simulink library "fc_vt_lib"  (Simulink 4.00)
undefined symbols (not defined in the file or in its folder): amb_tmp, compressor_mass_flow_map, compressor_pressure_map, compressor_temperature_rise_map, fc_air_comp_scale, fc_allowable_temp_rise, fc_cathode_pressure_drop, fc_cell_area, fc_cell_num, fc_comp_adeff_max, fc_comp_elec_eff, fc_comp_max_tmp, fc_comp_slpm_air_max, fc_comp_spd_max, fc_comp_voleff_max, fc_condenser_fan_flowrate, fc_condenser_fan_num, fc_condenser_fan_pwr_map, fc_condenser_frontal_area, fc_condenser_scale, fc_coolant_pump_flow_map, fc_coolant_pump_pwr_map, fc_cp_air, fc_cp_h2o_l, fc_cp_stack, fc_fuel_lhv, fc_k_air, fc_max_cathode_inlet_pressure, fc_min_cathode_inlet_pressure, fc_min_cell_volts, fc_min_sys_pwr_req, fc_min_temp_for_heat_rejection, fc_mw_air, fc_mw_h2, fc_mw_h20, fc_o2_percent, fc_p_amb, fc_polar_param_concentration, fc_polar_param_ohmic, fc_polar_param_ohmic_temp, fc_polar_param_ref_temp, fc_polar_param_tafel, fc_polar_param_temperature, fc_polar_param_voc, fc_radiator_bypass_delta_t, fc_radiator_fan_flowrate, fc_radiator_fan_num, fc_radiator_fan_pwr_map, fc_radiator_frontal_area, fc_radiator_no_fan_flowrate, fc_radiator_scale, fc_radiator_spd_ratio_fan_off, fc_radiator_spd_ratio_fan_on, fc_radiator_veh_spd_map, fc_reference_temperature, fc_rh_amb, fc_stack_i_map, fc_stack_pres_cor_map, fc_stack_pres_map, fc_stack_stoich_air_map ... (+10)
libraries: fc_vt_lib x54, simulink3 x9
(part 2 of 3)

== system fc_vt_lib/VT_FUELCELL_MODEL ==
  net Power Request : Inport  Port=1  LatchInput=off
  Constant2 : Constant  Value=fc_min_sys_pwr_req
  Demux : Demux  Outputs=6  BusSelectionMode=off
  If : If  NumInputs=2  IfExpression=u1<u2  ShowElse=on
  Mux2 : Mux  Orientation=left  Inputs=4
  Subsystem : Subsystem
      settings: RTWFcnNameOpts=Auto  RTWFileNameOpts=Auto
  Switch : Switch  Threshold=1
  Terminator : Terminator
  Water : Memory  Orientation=left  X0=0  InheritSampleTime=off
      settings: RTWStateStorageClass=Auto
  min_cell_voltage & net power gen : Subsystem  TreatAsAtomicUnit=on
      settings: RTWFcnNameOpts=Auto  RTWFileNameOpts=Auto
  min_system_power : Subsystem  TreatAsAtomicUnit=on
      settings: RTWFcnNameOpts=Auto  RTWFileNameOpts=Auto
  stack_temperature : Memory  Orientation=left  X0=fc_system_init_temp  InheritSampleTime=off
      settings: RTWStateStorageClass=Auto
  t_stack_coolant_in : Memory  Orientation=left  X0=fc_system_init_temp  InheritSampleTime=off
      settings: RTWStateStorageClass=Auto
  Net Power Gen : Outport  Port=1
  system_characteristics : Outport  Port=2
  wires:
  Demux/1 -> Net Power Gen/1
  Demux/2 -> stack_temperature/1
  Demux/4 -> t_stack_coolant_in/1
  Demux/5 -> Water/1
  t_stack_coolant_in/1 -> Mux2/2
  stack_temperature/1 -> Mux2/3
  Water/1 -> Mux2/4
  Subsystem/1(system_characteristics) -> system_characteristics/1
  Demux/6 -> Subsystem/1(In1)
  [net_power_request] -> If/1
  Constant2/1 -> If/2
  [net_power_request] -> Mux2/1
  Mux2/1 -> [system_input]
  [system_input] -> min_system_power/1(In1)
  If/2 -> min_cell_voltage & net power gen/Action
  [system_input] -> min_cell_voltage & net power gen/1(In1)
  If/1 -> min_system_power/Action
  min_system_power/1(system_characteristics) -> Switch/1
  min_system_power/2(enabled?) -> Switch/2
  min_cell_voltage & net power gen/1(Out1) -> Switch/3
  Switch/1 -> Demux/1
  net Power Request/1 -> [net_power_request]
  Demux/3 -> Terminator/1

== system fc_vt_lib/air_power ==
  note: [K]
  m_dot_air : Inport  Port=1  LatchInput=off
  eff_overall : Inport  Port=2  LatchInput=off
  pressure : Inport  Port=3  LatchInput=off
  Constant : Constant  Value=amb_tmp
  Constant1 : Constant  Value=fc_k_air
  Constant2 : Constant  Value=fc_k_air
  Constant3 : Constant  Value=1
  Constant5 : Constant  Value=1
  Constant6 : Constant  Value=fc_comp_elec_eff
  Cp Air : fc_vt_lib/Cp Water_Vapor
      settings: RTWFcnNameOpts=Auto  RTWFileNameOpts=Auto
  Math Function : Math  Operator=pow  OutputSignalType=auto
  Product : Product  Inputs=4  Multiplication=Element-wise(.*)  SaturateOnIntegerOverflow=on
  Product1 : Product  Inputs=*/  Multiplication=Element-wise(.*)  SaturateOnIntegerOverflow=on
  Product2 : Product  Inputs=*//  Multiplication=Element-wise(.*)  SaturateOnIntegerOverflow=on
  Sum : Sum  Inputs=|+-  SaturateOnIntegerOverflow=on
  Sum1 : Sum  Inputs=|+-  SaturateOnIntegerOverflow=on
  Sum2 : Sum  Inputs=|++  SaturateOnIntegerOverflow=on
  const : Constant  Value=273.15
  Out1 : Outport  Port=1
  wires:
  Cp Air/1 -> Product/2
  Product2/1 -> Out1/1
  eff_overall/1 -> Product2/3
  Constant6/1 -> Product2/2
  Product/1 -> Product2/1
  Sum1/1 -> Product/4
  Math Function/1 -> Sum1/1
  Constant5/1 -> Sum1/2
  Product1/1 -> Math Function/2
  pressure/1 -> Math Function/1
  Constant2/1 -> Product1/2
  Sum/1 -> Product1/1
  Constant3/1 -> Sum/2
  Constant1/1 -> Sum/1
  m_dot_air/1 -> Product/1
  Sum2/1 -> Cp Air/1, Product/3
  Constant/1 -> Sum2/2
  const/1 -> Sum2/1

== system fc_vt_lib/h2W ==
  temp : Inport  Port=1  LatchInput=off
  pressure (atm) : Inport  Port=2  LatchInput=off
  rh : Inport  Port=3  LatchInput=off
  1=air;  2=h2 : Inport  Port=4  LatchInput=off
  Constant : Constant  Value=fc_mw_h20
  Constant1 : Constant  Value=fc_mw_air
  Constant2 : Constant  Value=fc_mw_h2
  Product : Product  Inputs=*/*/  Multiplication=Element-wise(.*)  SaturateOnIntegerOverflow=on
  Product1 : Product  Inputs=2  Multiplication=Element-wise(.*)  SaturateOnIntegerOverflow=on
  Psat : fc_vt_lib/Psat
      settings: RTWFcnNameOpts=Auto  RTWFileNameOpts=Auto
  Sum : Sum  Inputs=-+  SaturateOnIntegerOverflow=on
  Switch : Switch  Threshold=2
  atm --> kPa : Gain  Gain=101.325  Multiplication=Element-wise(K.*u)  SaturateOnIntegerOverflow=on
  w : Outport  Port=1
  wires:
  Constant/1 -> Product/1
  temp/1 -> Psat/1
  Psat/1 -> Product1/1
  pressure (atm)/1 -> atm --> kPa/1
  rh/1 -> Product1/2
  Product1/1 -> Sum/1, Product/3
  Sum/1 -> Product/4
  Constant2/1 -> Switch/1
  1=air;  2=h2/1 -> Switch/2
  Constant1/1 -> Switch/3
  Switch/1 -> Product/2
  Product/1 -> w/1
  atm --> kPa/1 -> Sum/2

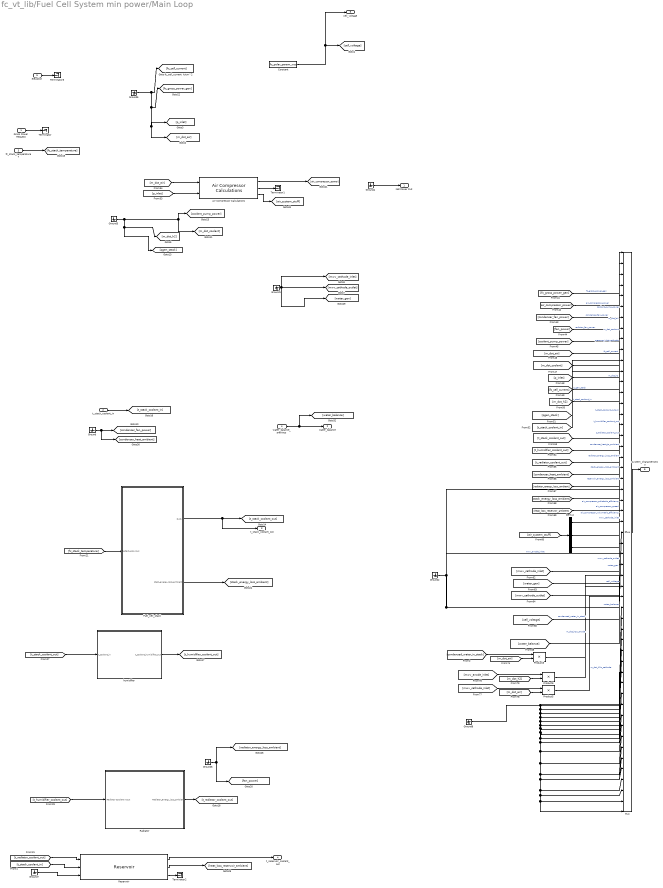
== system fc_vt_lib/Fuel Cell System min power/Main Loop ==
  Gross Power Request : Inport  Port=1  LatchInput=off
  t_stack_coolant_in : Inport  Port=2  LatchInput=off
  fc_stack_temperature7 : Inport  Port=3  LatchInput=off
  water_balance_previous : Inport  Port=4  LatchInput=off
  elevation : Inport  Port=5  LatchInput=off
  Air Compressor Calculations : fc_vt_lib/Main Loop/Air Compressor Calculations
      settings: RTWFcnNameOpts=Auto  RTWFileNameOpts=Auto
  Constant : Constant  Value=fc_polar_param_voc
  Demux : Demux  Outputs=3  BusSelectionMode=off
  Fuel_cell_stack : Subsystem  AncestorBlock=fc_vt_lib/Fuel Cell System min power/Main Loop/Fuel_cell_stack
      settings: RTWFcnNameOpts=Auto  RTWFileNameOpts=Auto
  Ground{,1..8} (9 alike) : Ground
  Mux : Mux  Inputs=53
  Product3 : Product  Inputs=2  Multiplication=Element-wise(.*)  SaturateOnIntegerOverflow=on
  Product5 : Product  Inputs=2  Multiplication=Element-wise(.*)  SaturateOnIntegerOverflow=on
  Product6 : Product  Inputs=2  Multiplication=Element-wise(.*)  SaturateOnIntegerOverflow=on
  Radiator : Subsystem  AncestorBlock=fc_vt_lib/Fuel Cell System min power/Main Loop/Radiator
      settings: RTWFcnNameOpts=Auto  RTWFileNameOpts=Auto
  Reservoir : fc_vt_lib/Main Loop/Reservoir
      settings: RTWFcnNameOpts=Auto  RTWFileNameOpts=Auto
  Terminator{,1..3} (4 alike) : Terminator
  humidifier : Subsystem  AncestorBlock=fc_vt_lib/Fuel Cell System min power/Main Loop/humidifier
      settings: RTWFcnNameOpts=Auto  RTWFileNameOpts=Auto
  Net Power Out : Outport  Port=1
  water_balance : Outport  Port=2
  t_stack_coolant_out : Outport  Port=3
  t_reservoir_coolant_out : Outport  Port=4
  cell_voltage : Outport  Port=5
  system_characteristics : Outport  Port=6
  wires:
  Air Compressor Calculations/2 -> Terminator1/1
  Ground3/1 -> [m_dot_coolant], [coolant_pump_power], [m_dot_h2], [qgen_stack]
  Ground4/1 -> Net Power Out/1
  [water_balance] -> Mux/30  "water_balance"
  [cell_voltage] -> Mux/28  "cell_voltage"
  Ground2/1 -> Mux/23, Mux/27, Mux/29  "mwv_anode_inlet"
  [mwv_cathode_inlet] -> Mux/24  "mwv_cathode_inlet"
  [water_gen] -> Mux/25  "water_gen"
  [mwv_cathode_outlet] -> Mux/26  "mwv_cathode_outlet"
  t_stack_coolant_in/1 -> [t_stack_coolant_in]
  fc_stack_temperature7/1 -> [fc_stack_temperature]
  [t_humidifier_coolant_out] -> Radiator/1(Radiator Coolant Input)
  Constant/1 -> [cell_voltage], cell_voltage/1
  Ground1/1 -> [mwv_cathode_inlet], [mwv_cathode_outlet], [water_gen]
  [t_radiator_coolant_out] -> Reservoir/1
  Reservoir/1 -> t_reservoir_coolant_out/1
  [t_stack_coolant_out] -> humidifier/1(t_coolant_in)
  humidifier/1(t_coolant_humidifier_out) -> [t_humidifier_coolant_out]
  [fc_stack_temperature] -> Fuel_cell_stack/1(t_stack_previous)
  Fuel_cell_stack/1(Out1) -> t_stack_coolant_out/1, [t_stack_coolant_out]
  Fuel_cell_stack/2(stack_energy_loss_ambient) -> [stack_energy_loss_ambient]
  Reservoir/2 -> [heat_loss_reservoir_ambient]
  Demux/3 -> Mux/22  "air_compressor_volumetric_efficiency"
  Demux/2 -> Mux/21  "air_compressor_adiabatic_efficiency"
  Demux/1 -> Mux/20  "air_compressor_speed"
  [heat_loss_reservoir_ambient] -> Mux/19  "reservoir_energy_loss_ambient"
  [stack_energy_loss_ambient] -> Mux/18  "stack_energy_loss_ambient"
  [radiator_energy_loss_ambient] -> Mux/17  "radiator_energy_loss_ambient"
  [condenser_heat_ambient] -> Mux/16  "condenser_heat_to_ambient"
  [t_radiator_coolant_out] -> Mux/15  "t_radiator_coolant_out"
  [t_humidifier_coolant_out] -> Mux/14  "t_humidifier_coolant_out"
  [t_stack_coolant_out] -> Mux/13  "t_stack_coolant_output"
  [t_stack_coolant_in] -> Mux/12  "t_stack_coolant_in"
  [qgen_stack] -> Mux/11  "q_gen_stack"
  [m_dot_h2] -> Mux/10  "m_dot_h2"
  [fc_cell_current] -> Mux/9  "fc_cell_current"
  [p_inlet] -> Mux/8  "pressure_inlet_cathode"
  [m_dot_coolant] -> Mux/7  "m_dot_coolant"
  [m_dot_air] -> Mux/6  "m_dot_air"
  [coolant_pump_power] -> Mux/5  "coolant_pump_power"
  [fan_power] -> Mux/4  "radiator_fan_power"
  [condenser_fan_power] -> Mux/3  "condenser_fan_power"
  [air_compressor_power] -> Mux/2  "air_compressor_power"
  [fc_gross_power_gen] -> Mux/1  "fc_gross_power_gen"
  [air_system_stuff] -> Demux/1
  Mux/1 -> system_characteristics/1
  Ground/1 -> [condenser_fan_power], [condenser_heat_ambient]
  [p_inlet] -> Air Compressor Calculations/2
  [m_dot_air] -> Air Compressor Calculations/1
  Air Compressor Calculations/1 -> [air_compressor_power]
  Air Compressor Calculations/3 -> [air_system_stuff]
  Ground5/1 -> [fc_cell_current], [fc_gross_power_gen], [p_inlet], [m_dot_air]
  Gross Power Request/1 -> Terminator/1
  Ground6/1 -> [fan_power], [radiator_energy_loss_ambient]
  Radiator/1(Radiator_energy_loss_ambient) -> [t_radiator_coolant_out]
  Ground7/1 -> Reservoir/3
  [t_stack_coolant_in] -> Reservoir/2
  Reservoir/3 -> Terminator2/1
  water_balance_previous/1 -> water_balance/1, [water_balance]
  Product3/1 -> Mux/31  "condensed_water_in_stack"
  [mwv_cathode_inlet] -> Product5/1
  [m_dot_air] -> Product5/2
  [mwv_anode_inlet] -> Product6/1
  [m_dot_h2] -> Product6/2
  Product6/1 -> Mux/32  "m_dot_h2o_anode"
  Product5/1 -> Mux/33  "m_dot_h2o_cathode"
  [condensed_water_in_stack] -> Product3/1
  [m_dot_air] -> Product3/2
  Ground8/1 -> Mux/41, Mux/42, Mux/43, Mux/44, Mux/45, Mux/46, Mux/47, Mux/48, Mux/49, Mux/50, Mux/51, Mux/52, Mux/53, Mux/40, Mux/39, Mux/38, Mux/37, Mux/36, Mux/35, Mux/34
  elevation/1 -> Terminator3/1

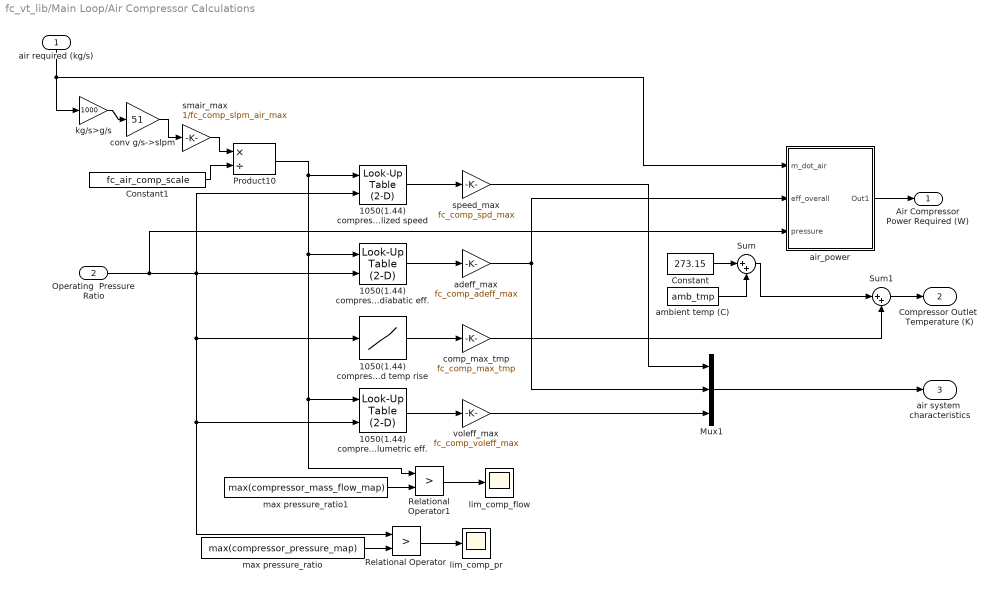
== system fc_vt_lib/Main Loop/Air Compressor Calculations ==
  " air required (kg/s)" : Inport  Orientation=down  Port=1  LatchInput=off
  Operating  Pressure Ratio : Inport  Port=2  LatchInput=off
  1050(1.44) compressor normalized adiabatic eff. : simulink3/Functions & Tables/Look-Up Table (2-D)  x=compressor_mass_flow_map  y=compressor_pressure_map  t=CC
  1050(1.44) compressor normalized speed : simulink3/Functions & Tables/Look-Up Table (2-D)  x=compressor_mass_flow_map  y=compressor_pressure_map  t=BB
  1050(1.44) compressor normalized temp rise : Lookup  InputValues=compressor_pressure_map  OutputValues=compressor_temperature_rise_map
  1050(1.44) compressor normalized volumetric eff. : simulink3/Functions & Tables/Look-Up Table (2-D)  x=compressor_mass_flow_map  y=compressor_pressure_map  t=DD
  Constant : Constant  Value=273.15
  Constant1 : Constant  Value=fc_air_comp_scale
  Mux1 : Mux  Inputs=3
  Product10 : Product  Inputs=*/  Multiplication=Element-wise(.*)  SaturateOnIntegerOverflow=on
  Relational Operator : RelationalOperator  Operator=>
  Relational Operator1 : RelationalOperator  Operator=>
  Sum : Sum  Inputs=|++  SaturateOnIntegerOverflow=on
  Sum1 : Sum  Inputs=|++  SaturateOnIntegerOverflow=on
  adeff_max : Gain  Gain=fc_comp_adeff_max  Multiplication=Element-wise(K.*u)  SaturateOnIntegerOverflow=on
  air_power : Subsystem  AncestorBlock=fc_vt_lib/air_power
      settings: RTWFcnNameOpts=Auto  RTWFileNameOpts=Auto
  ambient temp (C) : Constant  Value=amb_tmp
  comp_max_tmp : Gain  Gain=fc_comp_max_tmp  Multiplication=Element-wise(K.*u)  SaturateOnIntegerOverflow=on
  conv g/s->slpm : Gain  Gain=51  Multiplication=Element-wise(K.*u)  SaturateOnIntegerOverflow=on
  kg/s>g/s : Gain  Gain=1000  Multiplication=Element-wise(K.*u)  SaturateOnIntegerOverflow=on
  lim_comp_flow : Scope
      settings: TimeRange=auto  YMin=-5  YMax=5  SaveToWorkspace=off  LimitDataPoints=on  MaxDataPoints=5000
  lim_comp_pr : Scope
      settings: TimeRange=auto  YMin=-5  YMax=5  SaveToWorkspace=off  SaveName=ScopeData  LimitDataPoints=on  MaxDataPoints=5000
  max pressure_ratio : Constant  Value=max(compressor_pressure_map)
  max pressure_ratio1 : Constant  Value=max(compressor_mass_flow_map)
  smair_max : Gain  Gain=1/fc_comp_slpm_air_max  Multiplication=Element-wise(K.*u)  SaturateOnIntegerOverflow=on
  speed_max : Gain  Gain=fc_comp_spd_max  Multiplication=Element-wise(K.*u)  SaturateOnIntegerOverflow=on
  voleff_max : Gain  Gain=fc_comp_voleff_max  Multiplication=Element-wise(K.*u)  SaturateOnIntegerOverflow=on
  Air Compressor Power Required (W) : Outport  Port=1
  Compressor Outlet  Temperature (K) : Outport  Port=2
  air system  characteristics : Outport  Port=3
  wires:
  1050(1.44) compressor normalized volumetric eff./1 -> voleff_max/1
  comp_max_tmp/1 -> Sum1/2
  1050(1.44) compressor normalized temp rise/1 -> comp_max_tmp/1
  1050(1.44) compressor normalized adiabatic eff./1 -> adeff_max/1
  1050(1.44) compressor normalized speed/1 -> speed_max/1
  conv g/s->slpm/1 -> smair_max/1
  adeff_max/1 -> Mux1/2, air_power/2(eff_overall)
  " air required (kg/s)"/1 -> air_power/1(m_dot_air), kg/s>g/s/1
  Operating  Pressure Ratio/1 -> air_power/3(pressure), 1050(1.44) compressor normalized temp rise/1, 1050(1.44) compressor normalized volumetric eff./2, Relational Operator/1, 1050(1.44) compressor normalized speed/2, 1050(1.44) compressor normalized adiabatic eff./2
  Sum1/1 -> Compressor Outlet  Temperature (K)/1
  speed_max/1 -> Mux1/1
  voleff_max/1 -> Mux1/3
  Mux1/1 -> air system  characteristics/1
  air_power/1(Out1) -> Air Compressor Power Required (W)/1
  Constant/1 -> Sum/1
  ambient temp (C)/1 -> Sum/2
  Sum/1 -> Sum1/1
  max pressure_ratio/1 -> Relational Operator/2
  Relational Operator/1 -> lim_comp_pr/1
  max pressure_ratio1/1 -> Relational Operator1/2
  Relational Operator1/1 -> lim_comp_flow/1
  smair_max/1 -> Product10/1
  Product10/1 -> 1050(1.44) compressor normalized speed/1, 1050(1.44) compressor normalized adiabatic eff./1, 1050(1.44) compressor normalized volumetric eff./1, Relational Operator1/1
  Constant1/1 -> Product10/2
  kg/s>g/s/1 -> conv g/s->slpm/1

== system fc_vt_lib/Main Loop/Air Requirement Calculation ==
  Cell Voltage (V) : Inport  Port=1  LatchInput=off
  Fuel Cell Gross Power (W) : Inport  Port=2  LatchInput=off
  Stoic Rate Air : Inport  Port=3  LatchInput=off
  %-->fraction : Gain  Gain=1/100  Multiplication=Element-wise(K.*u)  SaturateOnIntegerOverflow=on
  4*F : Constant  Value=4*96485
  Molecular Weight of  Inlet Air (g/mole) : Subsystem
      settings: RTWFcnNameOpts=Auto  RTWFileNameOpts=Auto
  Molecular weight  of N2 (g/mole) : Constant  Value=28
  O2 Molecular Weight  (g/mole) : Constant  Value=32
  Product : Product  Inputs=**//  Multiplication=Element-wise(.*)  SaturateOnIntegerOverflow=on
  Product1 : Product  Inputs=*/*  Multiplication=Element-wise(.*)  SaturateOnIntegerOverflow=on
  g/s-->kg/s : Gain  Gain=1/1000  Multiplication=Element-wise(K.*u)  SaturateOnIntegerOverflow=on
  percent O2 in air : Constant  Value=fc_o2_percent
  m_dot_air kg/s : Outport  Port=1
  wires:
  O2 Molecular Weight  (g/mole)/1 -> Molecular Weight of  Inlet Air (g/mole)/2(In2)
  Stoic Rate Air/1 -> Product/1
  4*F/1 -> Product/4
  percent O2 in air/1 -> %-->fraction/1
  %-->fraction/1 -> Molecular Weight of  Inlet Air (g/mole)/1(In1), Product1/2
  Molecular Weight of  Inlet Air (g/mole)/1(Out1) -> Product1/3
  g/s-->kg/s/1 -> m_dot_air kg/s/1
  Product1/1 -> g/s-->kg/s/1
  Product/1 -> Product1/1
  Fuel Cell Gross Power (W)/1 -> Product/2
  Cell Voltage (V)/1 -> Product/3
  Molecular weight  of N2 (g/mole)/1 -> Molecular Weight of  Inlet Air (g/mole)/3(In3)

== system fc_vt_lib/Main Loop/Calculate the Required Water Flowrate for the Pump ==
  Stack gross Power Gen : Inport  Port=1  LatchInput=off
  Cell Voltage : Inport  Port=2  LatchInput=off
  2*F : Constant  Value=2*96485
  Deg C Rise : Constant  Value=fc_allowable_temp_rise
  J/g-->J/kg : Gain  Gain=1000  Multiplication=Element-wise(K.*u)  SaturateOnIntegerOverflow=on
  Lower Heating Value  Hydrogen (J/g) : Constant  Value=fc_fuel_lhv
  Molecular Weight H2  (kg/mole) : Constant  Value=2.02/1000
  Product : Product  Inputs=2  Multiplication=Element-wise(.*)  SaturateOnIntegerOverflow=on
  Product1 : Product  Inputs=*//  Multiplication=Element-wise(.*)  SaturateOnIntegerOverflow=on
  Specific Heat Water : Constant  Value=fc_cp_h2o_l
  Sum1 : Sum  Inputs=+-  SaturateOnIntegerOverflow=on
  m_dot_h2 : Product  Inputs=**//  Multiplication=Element-wise(.*)  SaturateOnIntegerOverflow=on
  coolant (kg/s) : Outport  Port=1
  m_dot_hydrogen : Outport  Port=2
  q_gen_stack : Outport  Port=3
  wires:
  Stack gross Power Gen/1 -> Sum1/2, m_dot_h2/1
  m_dot_h2/1 -> Product/1, m_dot_hydrogen/1
  Lower Heating Value  Hydrogen (J/g)/1 -> J/g-->J/kg/1
  Product/1 -> Sum1/1
  Sum1/1 -> Product1/1, q_gen_stack/1
  Deg C Rise/1 -> Product1/2
  Specific Heat Water/1 -> Product1/3
  Cell Voltage/1 -> m_dot_h2/3
  Product1/1 -> coolant (kg/s)/1
  Molecular Weight H2  (kg/mole)/1 -> m_dot_h2/2
  J/g-->J/kg/1 -> Product/2
  2*F/1 -> m_dot_h2/4

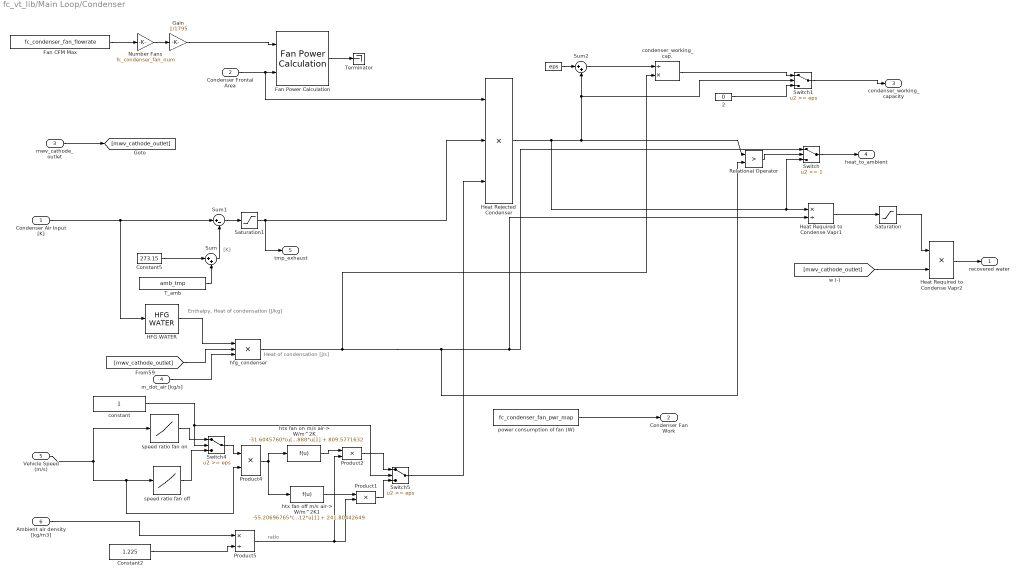
== system fc_vt_lib/Main Loop/Condenser ==
  note: [K]
  note: Enthalpy, Heat of condensation [J/kg]
  note: Heat of condensation [J/s]
  note: ratio
  Condenser Air Input [K] : Inport  Port=1  LatchInput=off
  Condenser Frontal Area : Inport  Port=2  LatchInput=off
  mwv_cathode_outlet : Inport  Port=3  LatchInput=off
  m_dot_air [kg/s] : Inport  Port=4  LatchInput=off
  Vehicle Speed (m/s) : Inport  Port=5  LatchInput=off
  Ambient air density [kg/m3] : Inport  Port=6  LatchInput=off
  " " : Constant  Value=eps
  " 2" : Constant  Value=0
  Constant2 : Constant  Value=1.225
  Constant5 : Constant  Value=273.15
  Fan CFM Max : Constant  Value=fc_condenser_fan_flowrate
  Fan Power Calculation : fc_vt_lib/Fan Power Calculation
      settings: RTWFcnNameOpts=Auto  RTWFileNameOpts=Auto
  Gain : Gain  Gain=1/1795  Multiplication=Element-wise(K.*u)  SaturateOnIntegerOverflow=on
  HFG WATER : fc_vt_lib/HFG WATER
      settings: RTWFcnNameOpts=Auto  RTWFileNameOpts=Auto
  Heat Rejected Condenser : Product  Inputs=***  Multiplication=Element-wise(.*)  SaturateOnIntegerOverflow=on
  Heat Required to Condense Vapr1 : Product  Inputs=*/  Multiplication=Element-wise(.*)  SaturateOnIntegerOverflow=on
  Heat Required to Condense Vapr2 : Product  Inputs=**  Multiplication=Element-wise(.*)  SaturateOnIntegerOverflow=on
  Number Fans : Gain  Gain=fc_condenser_fan_num  Multiplication=Element-wise(K.*u)  SaturateOnIntegerOverflow=on
  Product1 : Product  Inputs=**  Multiplication=Element-wise(.*)  SaturateOnIntegerOverflow=on
  Product2 : Product  Inputs=**  Multiplication=Element-wise(.*)  SaturateOnIntegerOverflow=on
  Product4 : Product  Inputs=**  Multiplication=Element-wise(.*)  SaturateOnIntegerOverflow=on
  Product5 : Product  Inputs=*/  Multiplication=Element-wise(.*)  SaturateOnIntegerOverflow=on
  Relational Operator : RelationalOperator  Operator=>
  Saturation : Saturate  UpperLimit=1  LowerLimit=0  LinearizeAsGain=on
  Saturation1 : Saturate  UpperLimit=inf  LowerLimit=0  LinearizeAsGain=on
  Sum : Sum  Inputs=|++  SaturateOnIntegerOverflow=on
  Sum1 : Sum  Inputs=|+-  SaturateOnIntegerOverflow=on
  Sum2 : Sum  Inputs=|++  SaturateOnIntegerOverflow=on
  Switch : Switch  Threshold=1
  Switch1 : Switch  Threshold=eps
  Switch4 : Switch  Threshold=eps
  Switch5 : Switch  Threshold=eps
  T_amb : Constant  Value=amb_tmp
  Terminator : Terminator
  condenser_working_cap. : Product  Inputs=/*  Multiplication=Element-wise(.*)  SaturateOnIntegerOverflow=on
  constant : Constant  Value=1
  hfg_condenser : Product  Inputs=***  Multiplication=Element-wise(.*)  SaturateOnIntegerOverflow=on
  htx fan off m/s air-> W/m^2K1 : Fcn  Expr=-55.20696765*(u[1]^2) + 920.65464912*u[1] + 241.80442649
  htx fan on m/s air-> W/m^2K : Fcn  Expr=-31.6045760*(u[1]^2) + 672.4946888*u[1] + 809.5771632
  power consumption of fan (W) : Constant  Value=fc_condenser_fan_pwr_map
  speed ratio fan off : Lookup  InputValues=fc_radiator_veh_spd_map  OutputValues=fc_radiator_spd_ratio_fan_off
  speed ratio fan on : Lookup  InputValues=fc_radiator_veh_spd_map  OutputValues=fc_radiator_spd_ratio_fan_on
  recovered water : Outport  Port=1
  Condenser Fan Work : Outport  Port=2
  condenser_working_capacity : Outport  Port=3
  heat_to_ambient : Outport  Port=4
  tmp_exhaust : Outport  Port=5
  wires:
  Saturation1/1 -> tmp_exhaust/1, Heat Rejected Condenser/2
  m_dot_air [kg/s]/1 -> hfg_condenser/3
  [mwv_cathode_outlet] -> hfg_condenser/2
  HFG WATER/1 -> hfg_condenser/1
  Fan CFM Max/1 -> Number Fans/1
  Number Fans/1 -> Gain/1
  Gain/1 -> Fan Power Calculation/1
  Condenser Air Input [K]/1 -> Sum1/1, HFG WATER/1
  Condenser Frontal Area/1 -> Fan Power Calculation/2, Heat Rejected Condenser/1
  mwv_cathode_outlet/1 -> [mwv_cathode_outlet]
  Sum1/1 -> Saturation1/1
  [mwv_cathode_outlet] -> Heat Required to Condense Vapr2/2
  hfg_condenser/1 -> condenser_working_cap./2, Relational Operator/2, Heat Required to Condense Vapr1/2, Switch/1
  Heat Rejected Condenser/1 -> Heat Required to Condense Vapr1/1, Switch/3, Relational Operator/1, Sum2/2, Switch1/2
  Relational Operator/1 -> Switch/2
  Switch/1 -> heat_to_ambient/1
  Heat Required to Condense Vapr1/1 -> Saturation/1
  Saturation/1 -> Heat Required to Condense Vapr2/1
  Heat Required to Condense Vapr2/1 -> recovered water/1
  Sum2/1 -> condenser_working_cap./1
  " "/1 -> Sum2/1
  Switch1/1 -> condenser_working_capacity/1
  condenser_working_cap./1 -> Switch1/1
  " 2"/1 -> Switch1/3
  Constant5/1 -> Sum/1
  T_amb/1 -> Sum/2
  Sum/1 -> Sum1/2
  speed ratio fan on/1 -> Switch4/1
  speed ratio fan off/1 -> Switch4/3
  Vehicle Speed (m/s)/1 -> speed ratio fan on/1, speed ratio fan off/1, Product4/2
  Switch4/1 -> Product4/1
  Product4/1 -> htx fan on m/s air-> W/m^2K/1, htx fan off m/s air-> W/m^2K1/1
  constant/1 -> Switch4/2, Switch5/2
  power consumption of fan (W)/1 -> Condenser Fan Work/1
  Switch5/1 -> Heat Rejected Condenser/3
  Fan Power Calculation/1 -> Terminator/1
  Constant2/1 -> Product5/2
  Product5/1 -> Product1/2, Product2/2
  Ambient air density [kg/m3]/1 -> Product5/1
  Product1/1 -> Switch5/3
  htx fan on m/s air-> W/m^2K/1 -> Product2/1
  Product2/1 -> Switch5/1
  htx fan off m/s air-> W/m^2K1/1 -> Product1/1

== system fc_vt_lib/Main Loop/Control Stratgegy for FC inlet cathode pressure ==
  Stack Current Density Operating Point : Inport  Port=1  LatchInput=off
  Stack Temperature : Inport  Port=2  LatchInput=off
  Ambient Pressure : Inport  Port=3  LatchInput=off
  Cathode Stoich Lookup : Lookup  InputValues=fc_stack_stoich_i_map  OutputValues=fc_stack_stoich_air_map
  Limit Pressure : Subsystem
      settings: RTWFcnNameOpts=Auto  RTWFileNameOpts=Auto
  Pressure Map Lookup ATM : Lookup  InputValues=fc_stack_i_map  OutputValues=fc_stack_pres_map
  Sum4 : Sum  Inputs=+|+  SaturateOnIntegerOverflow=on
  Temp Correction : Lookup  InputValues=fc_stack_temp_cor_map  OutputValues=fc_stack_pres_cor_map
  Pressure ATM : Outport  Port=1
  Air Stoich : Outport  Port=2
  wires:
  Temp Correction/1 -> Sum4/2
  Pressure Map Lookup ATM/1 -> Sum4/1
  Stack Current Density Operating Point/1 -> Pressure Map Lookup ATM/1, Cathode Stoich Lookup/1
  Stack Temperature/1 -> Temp Correction/1
  Limit Pressure/1(p req  limited) -> Pressure ATM/1
  Sum4/1 -> Limit Pressure/1(p req)
  Ambient Pressure/1 -> Limit Pressure/2(p amb)
  Cathode Stoich Lookup/1 -> Air Stoich/1

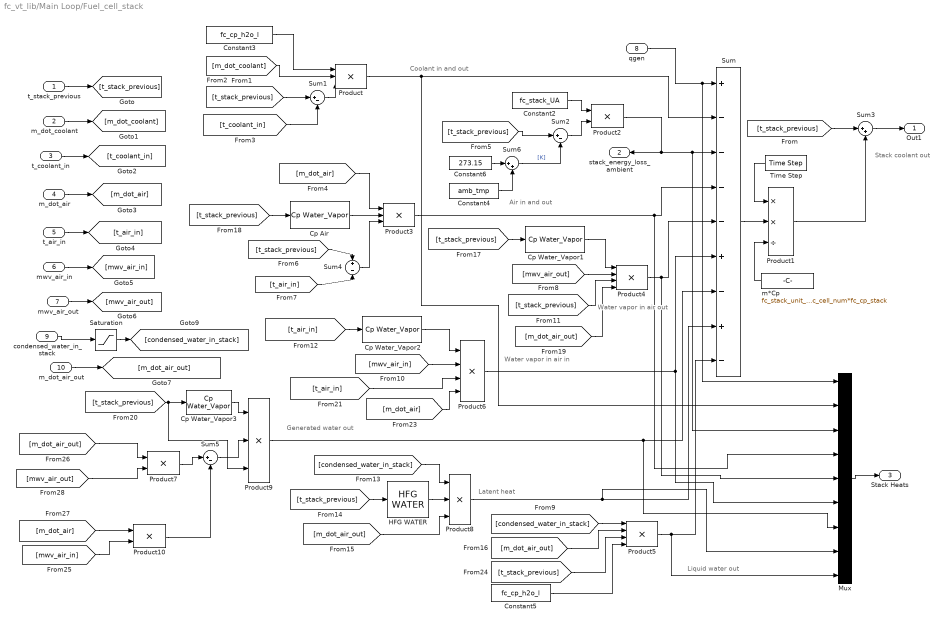
== system fc_vt_lib/Main Loop/Fuel_cell_stack ==
  note: Generated water out
  note: Coolant in and out
  note: Air in and out
  note: Water vapor
      | in air out
  note: Water vapor in air in
  note: Latent heat
  note: Liquid water out
  note: Stack coolant
      | out
  t_stack_previous : Inport  Port=1  LatchInput=off
  m_dot_coolant : Inport  Port=2  LatchInput=off
  t_coolant_in : Inport  Port=3  LatchInput=off
  m_dot_air : Inport  Port=4  LatchInput=off
  t_air_in : Inport  Port=5  LatchInput=off
  mwv_air_in : Inport  Port=6  LatchInput=off
  mwv_air_out : Inport  Port=7  LatchInput=off
  qgen : Inport  Port=8  LatchInput=off
  condensed_water_in_stack : Inport  Port=9  LatchInput=off
  m_dot_air_out : Inport  Port=10  LatchInput=off
  Constant2 : Constant  Value=fc_stack_UA
  Constant3 : Constant  Value=fc_cp_h2o_l
  Constant4 : Constant  Value=amb_tmp
  Constant5 : Constant  Value=fc_cp_h2o_l
  Constant6 : Constant  Value=273.15
  Cp Air : fc_vt_lib/Cp Water_Vapor
      settings: RTWFcnNameOpts=Auto  RTWFileNameOpts=Auto
  Cp Water_Vapor1 : fc_vt_lib/Cp Water_Vapor
      settings: RTWFcnNameOpts=Auto  RTWFileNameOpts=Auto
  Cp Water_Vapor2 : fc_vt_lib/Cp Water_Vapor
      settings: RTWFcnNameOpts=Auto  RTWFileNameOpts=Auto
  Cp Water_Vapor3 : fc_vt_lib/Cp Water_Vapor
      settings: RTWFcnNameOpts=Auto  RTWFileNameOpts=Auto
  HFG WATER : fc_vt_lib/HFG WATER
      settings: RTWFcnNameOpts=Auto  RTWFileNameOpts=Auto
  Mux : Mux  Inputs=9
  Product{,3,8..9} (4 alike) : Product  Inputs=3  Multiplication=Element-wise(.*)  SaturateOnIntegerOverflow=on
  Product1 : Product  Inputs=**/  Multiplication=Element-wise(.*)  SaturateOnIntegerOverflow=on
  Product10 : Product  Inputs=2  Multiplication=Element-wise(.*)  SaturateOnIntegerOverflow=on
  Product2 : Product  Inputs=2  Multiplication=Element-wise(.*)  SaturateOnIntegerOverflow=on
  Product4 : Product  Inputs=4  Multiplication=Element-wise(.*)  SaturateOnIntegerOverflow=on
  Product5 : Product  Inputs=4  Multiplication=Element-wise(.*)  SaturateOnIntegerOverflow=on
  Product6 : Product  Inputs=4  Multiplication=Element-wise(.*)  SaturateOnIntegerOverflow=on
  Product7 : Product  Inputs=2  Multiplication=Element-wise(.*)  SaturateOnIntegerOverflow=on
  Saturation : Saturate  UpperLimit=inf  LowerLimit=0  LinearizeAsGain=on
  Sum : Sum  Inputs=+----+-+-  SaturateOnIntegerOverflow=on
  Sum1 : Sum  Inputs=|+-  SaturateOnIntegerOverflow=on
  Sum2 : Sum  Inputs=|+-  SaturateOnIntegerOverflow=on
  Sum3 : Sum  Inputs=|++  SaturateOnIntegerOverflow=on
  Sum4 : Sum  Inputs=+-  SaturateOnIntegerOverflow=on
  Sum5 : Sum  Inputs=|+-  SaturateOnIntegerOverflow=on
  Sum6 : Sum  Inputs=|++  SaturateOnIntegerOverflow=on
  Time Step : fc_vt_lib/Time Step  Orientation=left
      settings: RTWFcnNameOpts=Auto  RTWFileNameOpts=Auto
  m*Cp : Constant  Orientation=left  Value=fc_stack_unit_mass*fc_cell_area*fc_cell_num*fc_cp_stack
  Out1 : Outport  Port=1
  stack_energy_loss_ambient : Outport  Orientation=left  Port=2
  Stack Heats : Outport  Port=3
  wires:
  Product5/1 -> Sum/9, Mux/9
  Constant5/1 -> Product5/4
  [t_stack_previous] -> Product5/3
  [m_dot_air_out] -> Product5/2
  [condensed_water_in_stack] -> Product5/1
  Product9/1 -> Sum/7, Mux/7
  Product4/1 -> Sum/5, Mux/5
  Product6/1 -> Sum/6, Mux/6
  Sum5/1 -> Product9/2
  Cp Water_Vapor3/1 -> Product9/1
  [t_stack_previous] -> Cp Water_Vapor3/1, Product9/3
  t_stack_previous/1 -> [t_stack_previous]
  m_dot_coolant/1 -> [m_dot_coolant]
  t_coolant_in/1 -> [t_coolant_in]
  m_dot_air/1 -> [m_dot_air]
  t_air_in/1 -> [t_air_in]
  mwv_air_in/1 -> [mwv_air_in]
  mwv_air_out/1 -> [mwv_air_out]
  qgen/1 -> Sum/1, Mux/1
  [t_stack_previous] -> Sum1/1
  [t_coolant_in] -> Sum1/2
  Constant3/1 -> Product/1
  [m_dot_coolant] -> Product/2
  Sum1/1 -> Product/3
  Product/1 -> Sum/2, Mux/2
  [t_stack_previous] -> Sum2/1
  Constant2/1 -> Product2/1
  Sum2/1 -> Product2/2
  [t_stack_previous] -> Sum4/1
  [t_air_in] -> Sum4/2
  [m_dot_air] -> Product3/1
  Cp Air/1 -> Product3/2
  Sum4/1 -> Product3/3
  Product2/1 -> stack_energy_loss_ambient/1, Sum/3, Mux/3
  Product3/1 -> Sum/4, Mux/4
  [t_stack_previous] -> Product4/3
  Cp Water_Vapor1/1 -> Product4/1
  m*Cp/1 -> Product1/3
  Time Step/1 -> Product1/1
  Sum/1 -> Product1/2
  Sum3/1 -> Out1/1
  Product1/1 -> Sum3/2
  [t_stack_previous] -> Sum3/1
  [t_stack_previous] -> Cp Water_Vapor1/1
  [t_stack_previous] -> Cp Air/1
  [m_dot_air_out] -> Product4/4
  [mwv_air_out] -> Product4/2
  [t_air_in] -> Product6/3
  Cp Water_Vapor2/1 -> Product6/1
  [t_air_in] -> Cp Water_Vapor2/1
  [m_dot_air] -> Product6/4
  [mwv_air_in] -> Product6/2
  condensed_water_in_stack/1 -> Saturation/1
  [t_stack_previous] -> HFG WATER/1
  [condensed_water_in_stack] -> Product8/1
  [m_dot_air_out] -> Product8/3
  Product8/1 -> Sum/8, Mux/8
  Constant6/1 -> Sum6/1
  Constant4/1 -> Sum6/2
  Sum6/1 -> Sum2/2  "[K]"
  Mux/1 -> Stack Heats/1
  m_dot_air_out/1 -> [m_dot_air_out]
  [m_dot_air_out] -> Product7/1
  [mwv_air_out] -> Product7/2
  Product7/1 -> Sum5/1
  [m_dot_air] -> Product10/1
  [mwv_air_in] -> Product10/2
  Product10/1 -> Sum5/2
  HFG WATER/1 -> Product8/2
  Saturation/1 -> [condensed_water_in_stack]

== system fc_vt_lib/Main Loop/Outlet Pressure Calculation ==
  Inlet Pressure : Inport  Port=1  LatchInput=off
  Sum2 : Sum  Inputs=+-  SaturateOnIntegerOverflow=on
  dim % : Constant  Value=fc_cathode_pressure_drop
  Outlet Pressure : Outport  Port=1
  Delta P : Outport  Port=2
  wires:
  Inlet Pressure/1 -> Sum2/1
  Sum2/1 -> Outlet Pressure/1
  dim %/1 -> Sum2/2, Delta P/1

== system fc_vt_lib/Main Loop/Partial Pressure Oxygen Operating Point Calculation1 ==
  note: Partial Pressure of Oxygen Operating Point Calculation
  Desired Cathode Humidity : Inport  Port=1  LatchInput=off
  "Stack Temp " : Inport  Port=2  LatchInput=off
  Inlet Pressure to Fuel Cell Stack : Inport  Port=3  LatchInput=off
  Air Stoic Rate : Inport  Port=4  LatchInput=off
  o2_percent : Inport  Port=5  LatchInput=off
  Outlet Pressure of Fuel Cell Stack : Inport  Port=6  LatchInput=off
  %-->fraction : Gain  Gain=1/100  Multiplication=Element-wise(K.*u)  SaturateOnIntegerOverflow=on
  Average Partial Pressure : Gain  Gain=1/2  Multiplication=Element-wise(K.*u)  SaturateOnIntegerOverflow=on
  Inlet Partial Pressure Calculation : Fcn  Expr=(u(3)-(u(2)*u(1)))*u(4)
  Mux : Mux  Inputs=4
  Mux1 : Mux  Inputs=6
  Mux2 : Mux  Inputs=3
  Outlet Partial Pressure Calculation : Fcn  Expr=((u(1)-u(2))-(u(3)*u(4)))*(u(6)*((u(5)-1)/u(5))/(1+u(6)*(((u(5)-1)/u(5))-1)))
  Psat : fc_vt_lib/Psat
      settings: RTWFcnNameOpts=Auto  RTWFileNameOpts=Auto
  Sum : Sum  Inputs=+|+  SaturateOnIntegerOverflow=on
  Sum1 : Sum  Inputs=+-  SaturateOnIntegerOverflow=on
  conv Pa->atm : Gain  Gain=1/101325  Multiplication=Element-wise(K.*u)  SaturateOnIntegerOverflow=on
  dim %1 : Constant  Value=fc_target_cathode_outlet_humidity
  O2 Avg  Partial Pressure : Outport  Port=1
  Partial Pressure Details : Outport  Port=2
  wires:
  Mux2/1 -> Partial Pressure Details/1
  %-->fraction/1 -> Mux1/6, Mux/4
  o2_percent/1 -> %-->fraction/1
  dim %1/1 -> Mux1/4
  Average Partial Pressure/1 -> O2 Avg  Partial Pressure/1
  Air Stoic Rate/1 -> Mux1/5
  Inlet Pressure to Fuel Cell Stack/1 -> Mux/3, Mux1/1, Sum1/1
  "Stack Temp "/1 -> Psat/1
  Sum/1 -> Average Partial Pressure/1
  Outlet Partial Pressure Calculation/1 -> Mux2/2, Sum/2
  Inlet Partial Pressure Calculation/1 -> Mux2/1, Sum/1
  Mux1/1 -> Outlet Partial Pressure Calculation/1
  Mux/1 -> Inlet Partial Pressure Calculation/1
  conv Pa->atm/1 -> Mux2/3, Mux1/3, Mux/2  "psat"
  Desired Cathode Humidity/1 -> Mux/1
  Psat/1 -> conv Pa->atm/1
  Outlet Pressure of Fuel Cell Stack/1 -> Sum1/2
  Sum1/1 -> Mux1/2

== system fc_vt_lib/Main Loop/Pump Coolant Power & Flow Rate ==
  requested  m_dot_coolant (kg/s) : Inport  Port=1  LatchInput=off
  Converwsion from  g/s->kg/s : Gain  Gain=1/1000  Multiplication=Element-wise(K.*u)  SaturateOnIntegerOverflow=on
  "Converwsion from  kg/s -> g/s" : Gain  Gain=1000  Multiplication=Element-wise(K.*u)  SaturateOnIntegerOverflow=on
  Limit Flowrate : Saturate  UpperLimit=max(fc_coolant_pump_flow_map)  LowerLimit=min(fc_coolant_pump_flow_map)  LinearizeAsGain=on
  Power (W) : Lookup  InputValues=fc_coolant_pump_flow_map  OutputValues=fc_coolant_pump_pwr_map
  Pump Power  Input (W) : Outport  Port=1
  actual  m_dot_coolant (kg/s) : Outport  Port=2
  wires:
  Power (W)/1 -> Pump Power  Input (W)/1
  requested  m_dot_coolant (kg/s)/1 -> "Converwsion from  kg/s -> g/s"/1
  Converwsion from  g/s->kg/s/1 -> actual  m_dot_coolant (kg/s)/1
  "Converwsion from  kg/s -> g/s"/1 -> Limit Flowrate/1
  Limit Flowrate/1 -> Power (W)/1, Converwsion from  g/s->kg/s/1

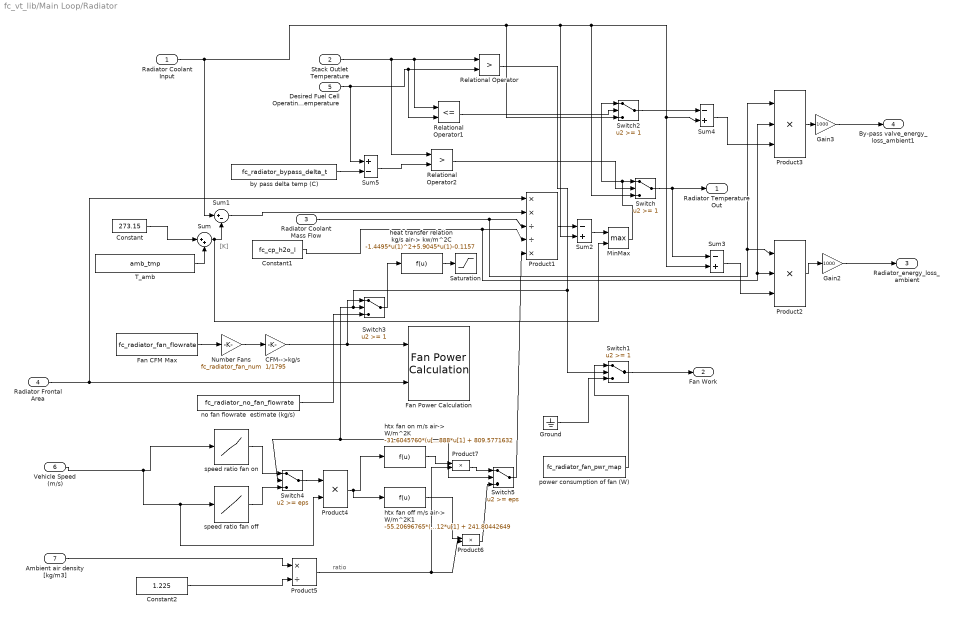
== system fc_vt_lib/Main Loop/Radiator ==
  note: [K]
  note: ratio
  Radiator Coolant Input : Inport  Port=1  LatchInput=off
  Stack Outlet Temperature : Inport  Port=2  LatchInput=off
  Radiator Coolant Mass Flow : Inport  Port=3  LatchInput=off
  Radiator Frontal Area : Inport  Port=4  LatchInput=off
  Desired Fuel Cell Operating Temperature : Inport  Port=5  LatchInput=off
  Vehicle Speed (m/s) : Inport  Port=6  LatchInput=off
  Ambient air density [kg/m3] : Inport  Port=7  LatchInput=off
  CFM-->kg/s : Gain  Gain=1/1795  Multiplication=Element-wise(K.*u)  SaturateOnIntegerOverflow=on
  Constant : Constant  Value=273.15
  Constant1 : Constant  Value=fc_cp_h2o_l
  Constant2 : Constant  Value=1.225
  Fan CFM Max : Constant  Value=fc_radiator_fan_flowrate
  Fan Power Calculation : fc_vt_lib/Fan Power Calculation
      settings: RTWFcnNameOpts=Auto  RTWFileNameOpts=Auto
  Gain2 : Gain  Gain=1000  Multiplication=Element-wise(K.*u)  SaturateOnIntegerOverflow=on
  Gain3 : Gain  Gain=1000  Multiplication=Element-wise(K.*u)  SaturateOnIntegerOverflow=on
  Ground : Ground
  MinMax : MinMax  Function=max  Inputs=2
  Number Fans : Gain  Gain=fc_radiator_fan_num  Multiplication=Element-wise(K.*u)  SaturateOnIntegerOverflow=on
  Product1 : Product  Inputs=**//*  Multiplication=Element-wise(.*)  SaturateOnIntegerOverflow=on
  Product2 : Product  Inputs=3  Multiplication=Element-wise(.*)  SaturateOnIntegerOverflow=on
  Product3 : Product  Inputs=3  Multiplication=Element-wise(.*)  SaturateOnIntegerOverflow=on
  Product4 : Product  Inputs=**  Multiplication=Element-wise(.*)  SaturateOnIntegerOverflow=on
  Product5 : Product  Inputs=*/  Multiplication=Element-wise(.*)  SaturateOnIntegerOverflow=on
  Product6 : Product  Inputs=**  Multiplication=Element-wise(.*)  SaturateOnIntegerOverflow=on
  Product7 : Product  Inputs=**  Multiplication=Element-wise(.*)  SaturateOnIntegerOverflow=on
  Relational Operator : RelationalOperator  Operator=>
  Relational Operator1 : RelationalOperator  Operator=<=
  Relational Operator2 : RelationalOperator  Operator=>
  Saturation : Saturate  UpperLimit=inf  LowerLimit=0  LinearizeAsGain=on
  Sum : Sum  Inputs=|++  SaturateOnIntegerOverflow=on
  Sum1 : Sum  Inputs=|+-  SaturateOnIntegerOverflow=on
  Sum2 : Sum  Inputs=-+  SaturateOnIntegerOverflow=on
  Sum3 : Sum  Inputs=-+  SaturateOnIntegerOverflow=on
  Sum4 : Sum  Inputs=-+  SaturateOnIntegerOverflow=on
  Sum5 : Sum  Inputs=+-  SaturateOnIntegerOverflow=on
  Switch{,1..3} (4 alike) : Switch  Threshold=1
  Switch4 : Switch  Threshold=eps
  Switch5 : Switch  Threshold=eps
  T_amb : Constant  Value=amb_tmp
  by pass delta temp (C) : Constant  Value=fc_radiator_bypass_delta_t
  heat transfer relation kg/s air-> kw/m^2C : Fcn  Expr=-1.4495*u(1)^2+5.9045*u(1)-0.1157
  htx fan off m/s air-> W/m^2K1 : Fcn  Expr=-55.20696765*(u[1]^2) + 920.65464912*u[1] + 241.80442649
  htx fan on m/s air-> W/m^2K : Fcn  Expr=-31.6045760*(u[1]^2) + 672.4946888*u[1] + 809.5771632
  no fan flowrate  estimate (kg/s) : Constant  Value=fc_radiator_no_fan_flowrate
  power consumption of fan (W) : Constant  Value=fc_radiator_fan_pwr_map
  speed ratio fan off : Lookup  InputValues=fc_radiator_veh_spd_map  OutputValues=fc_radiator_spd_ratio_fan_off
  speed ratio fan on : Lookup  InputValues=fc_radiator_veh_spd_map  OutputValues=fc_radiator_spd_ratio_fan_on
  Radiator Temperature Out : Outport  Port=1
  Fan Work : Outport  Port=2
  Radiator_energy_loss_ambient : Outport  Port=3
  By-pass valve_energy_loss_ambient1 : Outport  Port=4
  wires:
  Gain2/1 -> Radiator_energy_loss_ambient/1
  Fan CFM Max/1 -> Number Fans/1
  Number Fans/1 -> CFM-->kg/s/1
  Radiator Frontal Area/1 -> Product1/1, Fan Power Calculation/2
  CFM-->kg/s/1 -> Fan Power Calculation/1, Switch3/1
  Radiator Coolant Input/1 -> Sum1/1, Sum2/2, Switch/3, Sum3/2, Sum4/2, Switch2/3
  Sum1/1 -> Product1/2
  Product1/1 -> Sum2/1
  Radiator Coolant Mass Flow/1 -> Product1/3, Product2/1, Product3/1
  Constant1/1 -> Product1/4, Product3/2, Product2/2
  heat transfer relation kg/s air-> kw/m^2C/1 -> Saturation/1
  Switch/1 -> Sum3/1, Radiator Temperature Out/1
  Desired Fuel Cell Operating Temperature/1 -> Relational Operator/2, Relational Operator1/2, Sum5/1
  Relational Operator/1 -> Switch1/2, Switch3/2, Switch4/2, Switch5/2
  Sum3/1 -> Product2/3
  Product2/1 -> Gain2/1
  Switch1/1 -> Fan Work/1
  Ground/1 -> Switch1/3
  Stack Outlet Temperature/1 -> Relational Operator/1, Relational Operator1/1, Relational Operator2/1
  T_amb/1 -> Sum/2
  Sum/1 -> Sum1/2, MinMax/2
  Constant/1 -> Sum/1
  Relational Operator1/1 -> Switch2/2
  Switch2/1 -> Sum4/1
  Sum4/1 -> Product3/3
  Product3/1 -> Gain3/1
  Gain3/1 -> By-pass valve_energy_loss_ambient1/1
  Sum2/1 -> MinMax/1
  MinMax/1 -> Switch/1, Switch2/1
  Switch3/1 -> heat transfer relation kg/s air-> kw/m^2C/1
  no fan flowrate  estimate (kg/s)/1 -> Switch3/3
  Sum5/1 -> Relational Operator2/2
  by pass delta temp (C)/1 -> Sum5/2
  Relational Operator2/1 -> Switch/2
  speed ratio fan on/1 -> Switch4/1
  speed ratio fan off/1 -> Switch4/3
  Vehicle Speed (m/s)/1 -> speed ratio fan on/1, speed ratio fan off/1, Product4/2
  Switch4/1 -> Product4/1
  Product4/1 -> htx fan on m/s air-> W/m^2K/1, htx fan off m/s air-> W/m^2K1/1
  Switch5/1 -> Product1/5
  power consumption of fan (W)/1 -> Switch1/1
  Ambient air density [kg/m3]/1 -> Product5/1
  Constant2/1 -> Product5/2
  Product5/1 -> Product6/2, Product7/2
  htx fan off m/s air-> W/m^2K1/1 -> Product6/1
  Product6/1 -> Switch5/3
  htx fan on m/s air-> W/m^2K/1 -> Product7/1
  Product7/1 -> Switch5/1

== system fc_vt_lib/Main Loop/Reservoir ==
  t_reservoir_in : Inport  Port=1  LatchInput=off
  t_reservoir_previous : Inport  Port=2  LatchInput=off
  m_dot_coolant : Inport  Port=3  LatchInput=off
  Constant : Constant  Value=fc_system_coolant_capacity
  Constant1 : Constant  Value=fc_cp_h2o_l
  Constant2 : Constant  Value=0.00379
  Constant3 : Constant  Value=.001
  Constant4 : Constant  Value=amb_tmp
  Constant5 : Constant  Value=fc_sys_plumbing_htx_coef
  Constant6 : Constant  Value=273.15
  Constant8 : Constant  Value=fc_cp_h2o_l
  L-->gal : Gain  Gain=1/3.785  Multiplication=Element-wise(K.*u)  SaturateOnIntegerOverflow=on
  Product : Product  Inputs=***/  Multiplication=Element-wise(.*)  SaturateOnIntegerOverflow=on
  Product1 : Product  Inputs=*/  Multiplication=Element-wise(.*)  SaturateOnIntegerOverflow=on
  Product3 : Product  Inputs=3  Multiplication=Element-wise(.*)  SaturateOnIntegerOverflow=on
  Product4 : Product  Inputs=2  Multiplication=Element-wise(.*)  SaturateOnIntegerOverflow=on
  Product5 : Product  Inputs=2  Multiplication=Element-wise(.*)  SaturateOnIntegerOverflow=on
  Sum : Sum  Inputs=|+-  SaturateOnIntegerOverflow=on
  Sum1 : Sum  Inputs=|+-  SaturateOnIntegerOverflow=on
  Sum2 : Sum  Inputs=|-+  SaturateOnIntegerOverflow=on
  Sum3 : Sum  Inputs=|++  SaturateOnIntegerOverflow=on
  Sum4 : Sum  Inputs=|++  SaturateOnIntegerOverflow=on
  Time Step : fc_vt_lib/Time Step
      settings: RTWFcnNameOpts=Auto  RTWFileNameOpts=Auto
  t_reservoir_out : Outport  Port=1
  heat_loss_reservoir_ambient : Outport  Port=2
  thermal_capacity_coolant : Outport  Port=3
  wires:
  Constant/1 -> L-->gal/1
  Constant1/1 -> Product/2
  Constant2/1 -> Product/3
  Constant3/1 -> Product/4
  t_reservoir_in/1 -> Sum2/1, Sum/1
  Sum1/1 -> t_reservoir_out/1
  Constant8/1 -> Product3/1
  m_dot_coolant/1 -> Product3/2
  Sum2/1 -> Product3/3
  t_reservoir_previous/1 -> Sum2/2, [t_reservoir_previous]
  [t_reservoir_previous] -> Sum1/1
  Time Step/1 -> Product1/1
  Product/1 -> Product1/2
  Product1/1 -> thermal_capacity_coolant/1, Product4/1
  Sum/1 -> Product5/1
  Constant5/1 -> Product5/2
  Product5/1 -> heat_loss_reservoir_ambient/1, Sum3/1
  Product3/1 -> Sum3/2
  Sum3/1 -> Product4/2
  Product4/1 -> Sum1/2
  Constant4/1 -> Sum4/2
  Sum4/1 -> Sum/2
  Constant6/1 -> Sum4/1
  L-->gal/1 -> Product/1

== system fc_vt_lib/Main Loop/Subsystem ==
  Stack temperature [K] : Inport  Port=1  LatchInput=off
  cell voltage : Inport  Port=2  LatchInput=off
  Constant : Constant  Value=fc_reference_temperature
  Constant1 : Constant  Value=-1
  Faraday's constant : Constant  Value=96485
  Heat of reaction1 : fc_vt_lib/Heat of reaction
      settings: RTWFcnNameOpts=Auto  RTWFileNameOpts=Auto
  Product : Product  Inputs=4  Multiplication=Element-wise(.*)  SaturateOnIntegerOverflow=on
  Product1 : Product  Inputs=*/  Multiplication=Element-wise(.*)  SaturateOnIntegerOverflow=on
  numer of electrons  involved in the reaction : Constant  Value=2
  Cell efficiency : Outport  Port=1
  wires:
  Product1/1 -> Cell efficiency/1
  Heat of reaction1/1 -> Product1/2
  cell voltage/1 -> Product/4
  Product/1 -> Product1/1
  Faraday's constant/1 -> Product/3
  numer of electrons  involved in the reaction/1 -> Product/2
  Constant1/1 -> Product/1
  Constant/1 -> Heat of reaction1/2
  Stack temperature [K]/1 -> Heat of reaction1/1

== system fc_vt_lib/Main Loop/Subsystem1 ==
  net power [W] : Inport  Port=1  LatchInput=off
  mass flow H2 [kg/s] : Inport  Port=2  LatchInput=off
  J/g-->J/kg : Gain  Gain=1000  Multiplication=Element-wise(K.*u)  SaturateOnIntegerOverflow=on
  Lower Heating Value  Hydrogen (J/g) : Constant  Value=fc_fuel_lhv
  Product : Product  Inputs=2  Multiplication=Element-wise(.*)  SaturateOnIntegerOverflow=on
  Product1 : Product  Inputs=*/  Multiplication=Element-wise(.*)  SaturateOnIntegerOverflow=on
  "system_efficiency " : Outport  Port=1
  wires:
  Lower Heating Value  Hydrogen (J/g)/1 -> J/g-->J/kg/1
  J/g-->J/kg/1 -> Product/2
  mass flow H2 [kg/s]/1 -> Product/1
  net power [W]/1 -> Product1/1
  Product/1 -> Product1/2
  Product1/1 -> "system_efficiency "/1

== system fc_vt_lib/Main Loop/Subsystem2 ==
  m_dot_air [kg/s] : Inport  Port=1  LatchInput=off
  Cathode outlet water [-] : Inport  Port=2  LatchInput=off
  recovered [kg/s- : Inport  Port=3  LatchInput=off
  pressure : Inport  Port=4  LatchInput=off
  temperature : Inport  Port=5  LatchInput=off
  "Enthalpy (hf), Look-Up Table" : Lookup  InputValues=[1.0 1.2 1.4 1.6 1.8 2.0]  OutputValues=[417.5 439.2 458.3 475.4 490.7 504.8]
  "Enthalpy (hg), Look-Up Table1" : Lookup  InputValues=[1.0 1.2 1.4 1.6 1.8 2.0]  OutputValues=[2673.8 2682.0 2688.9 2695.0 2700.4 2705.2]
  Enthalpy [kj/kg]  Look-Up Table (2-D) : Subsystem  mask(Lookup Table (2-D)){x=[1.0 1.2 1.4 1.6 1.8 2.0], y=[293 303 313 323 333 343 353 363], t=[84.0 125.8 167.6 209.4 251.2 293.1 335.0 377.0;84.0 125.8 167.6 209.4 251.3 293.1 335.0 377.0;84.1 125.9 167.6 209.4 251.3 293.1 335.1 377.1;84.1 125.9 167.7 209.5 251.3 293.2 335.1 377.1;84.1 125.9 167.7 209.5 251.3 293.2 335.1 377.1;84.1 125.9 167.7 209.5 251.3 293.2 335.1 377.1]}
      mask prompts: x "Row:"; y "Column:"; t "Table:"
      mask help: Performs 2-D linear interpolation of input values using the specified input/output table. Extrapolation is performed outside the table boundaries. The first dimension corresponds to the top (or left) input port.
      mask init:
      | [r,c]=size(t);
      | xt=reshape(x,prod(size(x)),1);
      | xi=xt(:,ones(1,c));
      | minx=min(x); maxx=max(x);
      | mint=min(min(t)); maxt=max(max(t));
      settings: RTWFcnNameOpts=Auto  RTWFileNameOpts=Auto
      mask Display: plot(double(xi),double(t),double([minx maxx]),double([mint mint]),double([minx minx]),double([mint maxt]))
  Product1 : Product  Inputs=2  Multiplication=Element-wise(.*)  SaturateOnIntegerOverflow=on
  Product2 : Product  Inputs=2  Multiplication=Element-wise(.*)  SaturateOnIntegerOverflow=on
  Product3 : Product  Inputs=*/  Multiplication=Element-wise(.*)  SaturateOnIntegerOverflow=on
  Saturation : Saturate  UpperLimit=1  LowerLimit=0  LinearizeAsGain=on
  Sum : Sum  Inputs=|-+  SaturateOnIntegerOverflow=on
  Sum1 : Sum  Inputs=|+-  SaturateOnIntegerOverflow=on
  Sum2 : Sum  Inputs=|+-  SaturateOnIntegerOverflow=on
  atm->bar : Gain  Gain=1.013  Multiplication=Element-wise(K.*u)  SaturateOnIntegerOverflow=on
  kW->W : Gain  Gain=1000  Multiplication=Element-wise(K.*u)  SaturateOnIntegerOverflow=on
  water loss [kg/s] : Outport  Port=1
  heat loss [W] : Outport  Port=2
  quality [-] : Outport  Port=3
  wires:
  m_dot_air [kg/s]/1 -> Product1/1
  Cathode outlet water [-]/1 -> Product1/2
  Sum/1 -> water loss [kg/s]/1, Product2/1
  recovered [kg/s-/1 -> Sum/2
  Product1/1 -> Sum/1
  temperature/1 -> Enthalpy [kj/kg]  Look-Up Table (2-D)/2(Cols)
  Enthalpy [kj/kg]  Look-Up Table (2-D)/1(Out1) -> Product2/2, Sum1/1
  "Enthalpy (hf), Look-Up Table"/1 -> Sum1/2, Sum2/1
  pressure/1 -> atm->bar/1
  atm->bar/1 -> Enthalpy [kj/kg]  Look-Up Table (2-D)/1(Rows), "Enthalpy (hf), Look-Up Table"/1, "Enthalpy (hg), Look-Up Table1"/1
  Sum1/1 -> Product3/1
  "Enthalpy (hg), Look-Up Table1"/1 -> Sum2/2
  Sum2/1 -> Product3/2
  Product3/1 -> Saturation/1
  Saturation/1 -> quality [-]/1
  Product2/1 -> kW->W/1
  kW->W/1 -> heat loss [W]/1

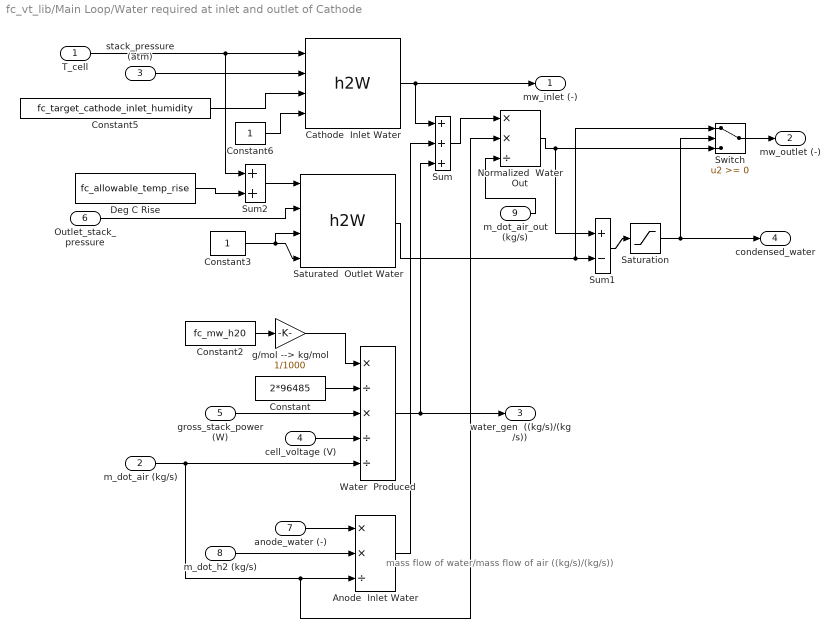
== system fc_vt_lib/Main Loop/Water required at inlet and outlet of Cathode ==
  note: mass flow of water/mass flow of air
      | ((kg/s)/(kg/s))
  T_cell : Inport  Port=1  LatchInput=off
  m_dot_air (kg/s) : Inport  Port=2  LatchInput=off
  stack_pressure (atm) : Inport  Port=3  LatchInput=off
  cell_voltage (V) : Inport  Port=4  LatchInput=off
  gross_stack_power (W) : Inport  Port=5  LatchInput=off
  Outlet_stack_pressure : Inport  Port=6  LatchInput=off
  anode_water (-) : Inport  Port=7  LatchInput=off
  m_dot_h2 (kg/s) : Inport  Port=8  LatchInput=off
  m_dot_air_out (kg/s) : Inport  Port=9  LatchInput=off
  "Anode  Inlet Water " : Product  Inputs=**/  Multiplication=Element-wise(.*)  SaturateOnIntegerOverflow=on
  Cathode  Inlet Water : fc_vt_lib/h2W
      settings: RTWFcnNameOpts=Auto  RTWFileNameOpts=Auto
  Constant : Constant  Value=2*96485
  Constant2 : Constant  Value=fc_mw_h20
  Constant3 : Constant  Value=1
  Constant5 : Constant  Value=fc_target_cathode_inlet_humidity
  Constant6 : Constant  Value=1
  Deg C Rise : Constant  Value=fc_allowable_temp_rise
  Normalized  Water Out : Product  Inputs=**/  Multiplication=Element-wise(.*)  SaturateOnIntegerOverflow=on
  Saturated  Outlet Water : fc_vt_lib/h2W
      settings: RTWFcnNameOpts=Auto  RTWFileNameOpts=Auto
  Saturation : Saturate  UpperLimit=inf  LowerLimit=-inf  LinearizeAsGain=on
  Sum : Sum  Inputs=+++  SaturateOnIntegerOverflow=on
  Sum1 : Sum  Inputs=+-  SaturateOnIntegerOverflow=on
  Sum2 : Sum  Inputs=++  SaturateOnIntegerOverflow=on
  Switch : Switch  Threshold=0
  Water  Produced : Product  Inputs=*/*//  Multiplication=Element-wise(.*)  SaturateOnIntegerOverflow=on
  g/mol --> kg/mol : Gain  Gain=1/1000  Multiplication=Element-wise(K.*u)  SaturateOnIntegerOverflow=on
  mw_inlet (-) : Outport  Port=1
  mw_outlet (-) : Outport  Port=2
  water_gen  ((kg/s)/(kg/s)) : Outport  Port=3
  condensed_water : Outport  Port=4
  wires:
  Saturated  Outlet Water/1 -> Switch/1, Sum1/2
  Constant3/1 -> Saturated  Outlet Water/4, Saturated  Outlet Water/3
  m_dot_air_out (kg/s)/1 -> Normalized  Water Out/3
  Sum/1 -> Normalized  Water Out/1
  g/mol --> kg/mol/1 -> Water  Produced/1
  Constant/1 -> Water  Produced/2
  Constant2/1 -> g/mol --> kg/mol/1
  Saturation/1 -> condensed_water/1, Switch/2
  Sum1/1 -> Saturation/1
  Normalized  Water Out/1 -> Switch/3, Sum1/1
  Switch/1 -> mw_outlet (-)/1
  Cathode  Inlet Water/1 -> Sum/1, mw_inlet (-)/1
  Outlet_stack_pressure/1 -> Saturated  Outlet Water/2
  m_dot_air (kg/s)/1 -> Normalized  Water Out/2, "Anode  Inlet Water "/3, Water  Produced/5
  cell_voltage (V)/1 -> Water  Produced/4
  gross_stack_power (W)/1 -> Water  Produced/3
  Constant6/1 -> Cathode  Inlet Water/4
  Constant5/1 -> Cathode  Inlet Water/3
  Water  Produced/1 -> Sum/3, water_gen  ((kg/s)/(kg/s))/1
  stack_pressure (atm)/1 -> Cathode  Inlet Water/2
  T_cell/1 -> Cathode  Inlet Water/1, Sum2/1
  anode_water (-)/1 -> "Anode  Inlet Water "/1
  m_dot_h2 (kg/s)/1 -> "Anode  Inlet Water "/2
  "Anode  Inlet Water "/1 -> Sum/2
  Sum2/1 -> Saturated  Outlet Water/1
  Deg C Rise/1 -> Sum2/2
